simulink model "model_Ster_Adaptacyjne_am"  (R2022a)
settings: Solver=FixedStepAuto  StartTime=0.0  StopTime=100  FixedStep=0.01  RelTol=1e-3
values from neighbouring files (symbols this model uses):
  am = 2    [Modified_MIT_skrypt_Ster_Adaptacyjne_am.m]    (also in skrypt_Ster_Adaptacyjne_am.m)
  gamma = gamma_vec(i)    [Modified_MIT_skrypt_Ster_Adaptacyjne_am.m]    (also in skrypt_Ster_Adaptacyjne.m; skrypt_Ster_Adaptacyjne_2_rzedu.m; skrypt_Ster_Adaptacyjne_am.m)
settings Model: Creator=marci  LastModifiedBy=marci

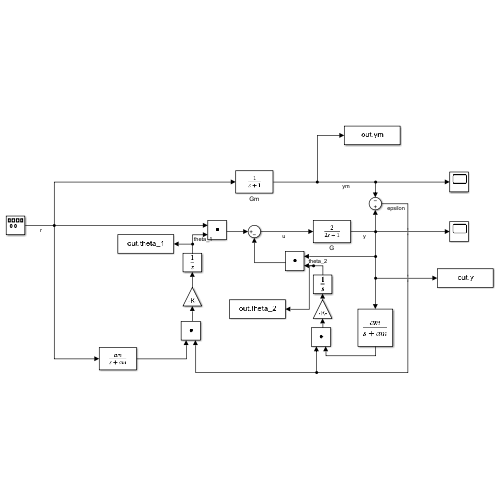
[thumbnail: Simulink's stored preview of the top-level diagram]
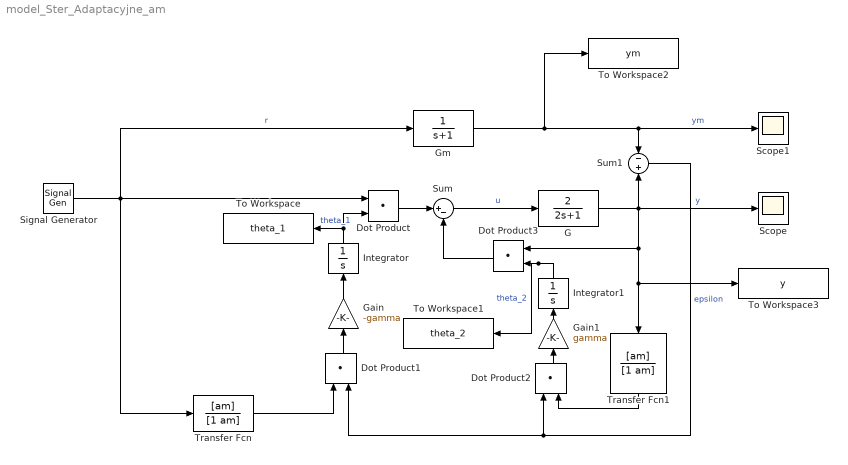
== system model_Ster_Adaptacyjne_am ==
  Dot Product{,1..3} (4 alike) : DotProduct  OutDataTypeStr=Inherit: Inherit via internal rule
  G : TransferFcn  Numerator=[2]  Denominator=[2 1]
  Gain : Gain  Gain=-gamma
  Gain1 : Gain  Gain=gamma
  Gm : TransferFcn  Denominator=[1 1]
  Integrator : Integrator
  Integrator1 : Integrator
  Scope : Scope
  Scope1 : Scope
  Signal Generator : SignalGenerator  WaveForm=square  Frequency=0.1
  Sum : Sum  Inputs=|+-
  Sum1 : Sum  Inputs=-+
  To Workspace : ToWorkspace  VariableName=theta_1  SaveFormat=Timeseries  SampleTime=-1
  To Workspace1 : ToWorkspace  VariableName=theta_2  SaveFormat=Timeseries  SampleTime=-1
  To Workspace2 : ToWorkspace  VariableName=ym  SaveFormat=Timeseries  SampleTime=-1
  To Workspace3 : ToWorkspace  VariableName=y  SaveFormat=Timeseries  SampleTime=-1
  Transfer Fcn : TransferFcn  Numerator=[am]  Denominator=[1 am]
  Transfer Fcn1 : TransferFcn  Numerator=[am]  Denominator=[1 am]
  wires:
  Signal Generator/1 -> Transfer Fcn/1, Gm/1, Dot Product/1  "r"
  Transfer Fcn/1 -> Dot Product1/1
  Dot Product1/1 -> Gain/1
  Gain/1 -> Integrator/1
  Integrator/1 -> To Workspace/1, Dot Product/2  "theta_1"
  Dot Product/1 -> Sum/1
  Dot Product3/1 -> Sum/2
  Dot Product2/1 -> Gain1/1
  Gain1/1 -> Integrator1/1
  Integrator1/1 -> To Workspace1/1, Dot Product3/2  "theta_2"
  Sum/1 -> G/1  "u"
  G/1 -> To Workspace3/1, Transfer Fcn1/1, Dot Product3/1, Scope/1, Sum1/2  "y"
  Gm/1 -> To Workspace2/1, Scope1/1, Sum1/1  "ym"
  Transfer Fcn1/1 -> Dot Product2/2
  Sum1/1 -> Dot Product1/2, Dot Product2/1  "epsilon"
